simulink model "main_slx"  (R2015b)
settings: Solver=FixedStepAuto  SolverMode=SingleTasking  StartTime=0.0  StopTime=15  FixedStep=0.008  RelTol=1e-3
undefined symbols (not defined in the file or in its folder): CR, LF, serial
libraries: instrumentlib x2
settings Model: Creator=Wasin  LastModifiedBy=Wasin
settings SolverCC: AutoInsertRateTranBlk=on  InsertRTBMode=Never (minimum delay)
settings DataIOCC: SaveFormat=Array
settings HardwareCC: ProdBitPerPointer=32  ProdLargestAtomicFloat=None  ProdIntDivRoundTo=Undefined  ProdEndianess=Unspecified  ProdWordSize=32  ProdHWDeviceType=32-bit Generic
settings GRTTargetCC: GeneratePreprocessorConditionals=Disable all
settings ConfigComp: CovModelRefEnable=Off

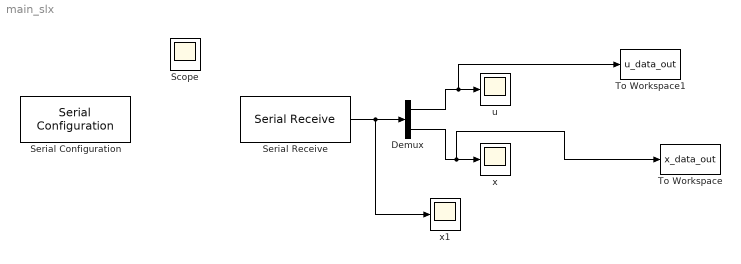
== system main_slx ==
  Demux : Demux  Outputs=2
  Serial Configuration : instrumentlib/Serial Configuration  Priority=-200000  ComPortMenu=<Please select a port...>  ComPort=COM5  ObjConstructor=serial('COM5');  BaudRate=115200  DataBits=8  Parity=none  StopBits=1  FlowControl=none  Timeout=4  ByteOrder=LittleEndian
  Serial Receive : instrumentlib/Serial Receive  ComPortMenu=<Please select a port...>  ComPort=COM5  ObjConstructor=serial('COM5');  Terminator=CR/LF ('\r\n')  DataSize="[1  2]"  DataType=int16  EnableBlockingMode=on  ActionDataUnavailable=Output last received value  CustomValue=0  SampleTime=0.008
  To Workspace : ToWorkspace  VariableName=x_data_out  SaveFormat=Structure With Time  SampleTime=-1
  To Workspace1 : ToWorkspace  VariableName=u_data_out  SaveFormat=Structure With Time  SampleTime=-1
  u : Scope
  x : Scope
  x1 : Scope
  Scope : Scope
  wires:
  Serial Receive/1 -> x1/1, Demux/1
  Demux/1 -> To Workspace1/1, u/1
  Demux/2 -> To Workspace/1, x/1
